simulink model "Ph3_2Lvl_SVPWM_Comparison"  (R2022b)
settings: Solver=FixedStepDiscrete  StartTime=0.0  StopTime=1.2  FixedStep=1/(100*9600)  RelTol=1e-3
libraries: spsSeriesRLCBranchLib x15, spsRMSLib x10, spsMosfetLib x6, simulink x5, spsThreePhaseVIMeasurementLib x2, spsDCVoltageSourceLib x1, spsGroundLib x1, spsVoltageMeasurementLib x1, sps_lib x1
settings Model: Creator=XIAO  LastModifiedBy=XIAO
settings SolverCC: AutoInsertRateTranBlk=on
settings DataIOCC: ReturnWorkspaceOutputs=off  LoggingToFile=on

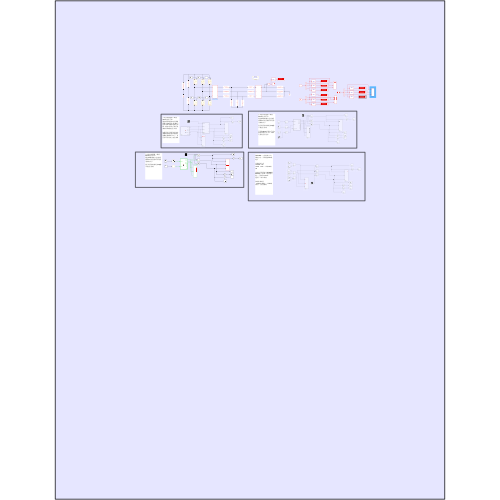
[thumbnail: Simulink's stored preview of the top-level diagram]
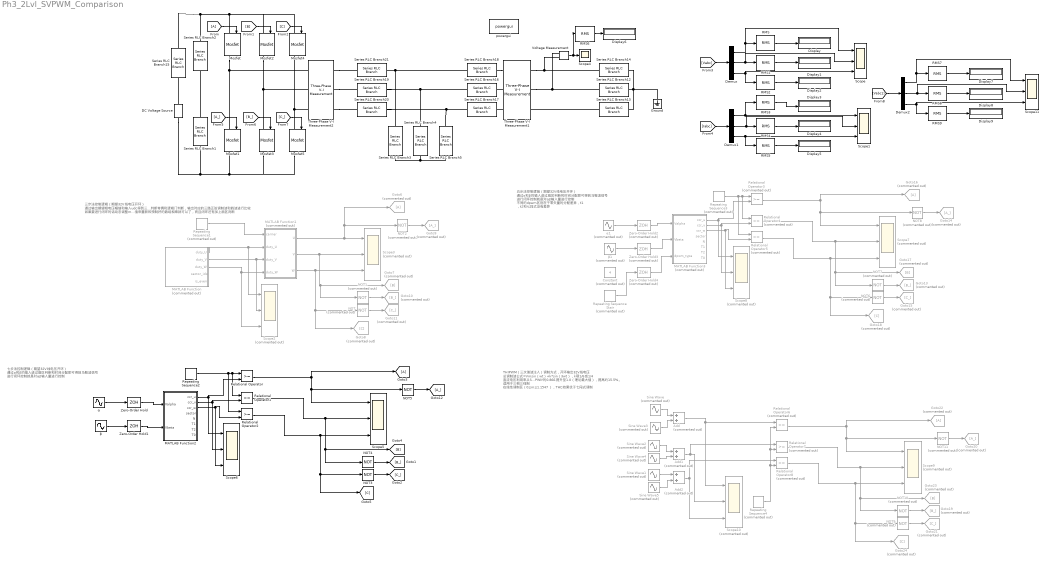
== system Ph3_2Lvl_SVPWM_Comparison ==
  note: 三步法控制逻辑（期望32V线电压开环）
      | 通过输出期望相电压幅值和输入udc得到三组数组，然后判断奇偶和逻辑门判断，输出对应的三路正弦调制波和载波进行比较
      |
      | 如果要进行闭环的话动态调整m值来重新和预制好的数组相乘就可以了，而且闭环还有加上扇区判断
  note: 七步法控制逻辑（期望32V线电压开环）
      | 通过α和β的输入进过扇区判断和时间分配即可得到马鞍波信号
      |
      | 进行闭环控制就是对αβ输入量进行控制
  note: 五步法控制逻辑（期望32V线电压开环）
      | 通过α和β的输入进过扇区判断和时间分配即可得到马鞍波信号
      |
      | 进行闭环控制就是对αβ输入量进行控制
      |
      | 不同的dpwm区别在于零矢量的分配差异，t1 ，t2和七段式没有差异
  note: THIPWM（三次谐波注入）调制方式，开环输出32V线电压
      |
      | 总调制波公式=Vmsin（wt）+k*sin（3wt），k取1/6或1/4
      |
      | 直流电压利用率从SPWM的0.866提升至1.0（理论最大值），提高约15.5%。
      | 适用于三相三线制
      |
      | 在线性调制区（0≤m≤1.1547），THD效果优于七段式调制
  Add : Sum  Commented=on
  Add1 : Sum  Commented=on
  Add2 : Sum  Commented=on
  Constant : Constant  Commented=on  Value=4
  DC Voltage Source : spsDCVoltageSourceLib/DC Voltage Source  Amplitude=60  Measurements=None
  Demux : Demux  Outputs=3
  Demux1 : Demux  Outputs=3
  Demux2 : Demux  Outputs=3
  Display{,1..9} (10 alike) : Display
  From : From
  Goto10 : Goto  Commented=on  GotoTag=B_
  Goto11 : Goto  Commented=on  GotoTag=C_
  Goto13 : Goto  Commented=on  GotoTag=B_
  Goto14 : Goto  Commented=on  GotoTag=A_
  Goto15 : Goto  Commented=on  GotoTag=C_
  Goto16 : Goto  Commented=on
  Goto17 : Goto  Commented=on  GotoTag=B
  Goto18 : Goto  Commented=on  GotoTag=C
  Goto19 : Goto  Commented=on  GotoTag=B_
  Goto20 : Goto  Commented=on  GotoTag=A_
  Goto21 : Goto  Commented=on  GotoTag=C_
  Goto22 : Goto  Commented=on
  Goto23 : Goto  Commented=on  GotoTag=B
  Goto24 : Goto  Commented=on  GotoTag=C
  Goto3 : Goto
  Goto6 : Goto  Commented=on
  Goto7 : Goto  Commented=on  GotoTag=B
  Goto8 : Goto  Commented=on  GotoTag=C
  Goto9 : Goto  Commented=on  GotoTag=A_
  Ground : spsGroundLib/Ground  LConnTagsString=a
  MATLAB Function : MATLAB Function  Commented=on  TreatAsAtomicUnit=on  SystemSampleTime=1/9600
  MATLAB Function1 : MATLAB Function  Commented=on  TreatAsAtomicUnit=on  SystemSampleTime=1/(100*9600)
  MATLAB Function2 : MATLAB Function  TreatAsAtomicUnit=on
  MATLAB Function3 : MATLAB Function  Commented=on  TreatAsAtomicUnit=on
  Mosfet{,1..5} (6 alike) : spsMosfetLib/Mosfet  Ron=0.1  Lon=0  Rd=0.01  Vfd=0  IC=0  Rs=1e5  Cs=inf  Measurements=on
  NOT{,1..2,6..11} (9 alike) : Logic  Commented=on  Operator=NOT  IconShape=distinctive  AllPortsSameDT=off  OutDataTypeStr=boolean
  NOT3 : Logic  Operator=NOT  IconShape=distinctive  AllPortsSameDT=off  OutDataTypeStr=boolean
  NOT4 : Logic  Operator=NOT  IconShape=distinctive  AllPortsSameDT=off  OutDataTypeStr=boolean
  NOT5 : Logic  Operator=NOT  IconShape=distinctive  AllPortsSameDT=off  OutDataTypeStr=boolean
  RMS{,1..9} (10 alike) : spsRMSLib/RMS  TrueRMS=on  Freq=50  RMSInit=120  Ts=1/(100*9600)
  Relational Operator : RelationalOperator  OutDataTypeStr=boolean  RndMeth=Simplest  InputSameDT=off
  Relational Operator1 : RelationalOperator  OutDataTypeStr=boolean  RndMeth=Simplest  InputSameDT=off
  Relational Operator2 : RelationalOperator  OutDataTypeStr=boolean  RndMeth=Simplest  InputSameDT=off
  Relational Operator{3..8} (6 alike) : RelationalOperator  Commented=on  OutDataTypeStr=boolean  RndMeth=Simplest  InputSameDT=off
  Repeating Sequence Stair : simulink/Sources/Repeating Sequence Stair  Commented=on  OutValues=[1 2 3 4 5 6]  tsamp=0.2  OutMin=[]  OutMax=[]  OutDataTypeStr=double  OutputDataTypeScalingMode=double  OutDataType=fixdt(0,8)  ConRadixGroup=Best Precision: Vector-wise  OutScaling=2^-12
  Repeating Sequence1 : simulink/Sources/Repeating Sequence  Commented=on  rep_seq_t=[0, 1/9600]  rep_seq_y=[0,1]
  Repeating Sequence2 : simulink/Sources/Repeating Sequence  rep_seq_t=[0, 1/20000, 1/10000]  rep_seq_y=[0,8500,0]
  Repeating Sequence3 : simulink/Sources/Repeating Sequence  Commented=on  rep_seq_t=[0, 1/20000, 1/10000]  rep_seq_y=[0,8500,0]
  Repeating Sequence4 : simulink/Sources/Repeating Sequence  Commented=on  rep_seq_t=[0, 1/20000, 1/10000]  rep_seq_y=[-1,1,-1]
  Scope{,1,5..6,11} (5 alike) : Scope  NumInputPorts=3
  Scope{2..3,7..10} (6 alike) : Scope  Commented=on  NumInputPorts=3
  Scope4 : Scope
  Series RLC Branch1 : spsSeriesRLCBranchLib/Series RLC Branch  LConnTagsString=__new0  RConnTagsString=__new0  BranchType=C  Resistance=1  Inductance=1e-3  SetiL0=off  InitialCurrent=0  Capacitance=1000e-6  Setx0=off  InitialVoltage=0  Measurements=None
  Series RLC Branch12 : spsSeriesRLCBranchLib/Series RLC Branch  LConnTagsString=__new0  RConnTagsString=__new0  BranchType=R  Resistance=200  Inductance=1e-3  SetiL0=off  InitialCurrent=0  Capacitance=1000e-6  Setx0=off  InitialVoltage=0  Measurements=None
  Series RLC Branch13 : spsSeriesRLCBranchLib/Series RLC Branch  LConnTagsString=__new0  RConnTagsString=__new0  BranchType=R  Resistance=200  Inductance=1e-3  SetiL0=off  InitialCurrent=0  Capacitance=1000e-6  Setx0=off  InitialVoltage=0  Measurements=None
  Series RLC Branch14 : spsSeriesRLCBranchLib/Series RLC Branch  LConnTagsString=__new0  RConnTagsString=__new0  BranchType=R  Resistance=200  Inductance=1e-3  SetiL0=off  InitialCurrent=0  Capacitance=1000e-6  Setx0=off  InitialVoltage=0  Measurements=None
  Series RLC Branch15 : spsSeriesRLCBranchLib/Series RLC Branch  LConnTagsString=__new0  RConnTagsString=__new0  BranchType=R  Resistance=0.1  Inductance=1e-3  SetiL0=off  InitialCurrent=0  Capacitance=1000e-6  Setx0=off  InitialVoltage=0  Measurements=None
  Series RLC Branch16 : spsSeriesRLCBranchLib/Series RLC Branch  LConnTagsString=__new0  RConnTagsString=__new0  BranchType=L  Resistance=1  Inductance=120.e-6  SetiL0=off  InitialCurrent=0  Capacitance=1000e-6  Setx0=off  InitialVoltage=0  Measurements=None
  Series RLC Branch17 : spsSeriesRLCBranchLib/Series RLC Branch  LConnTagsString=__new0  RConnTagsString=__new0  BranchType=L  Resistance=1  Inductance=120e-6  SetiL0=off  InitialCurrent=0  Capacitance=1000e-6  Setx0=off  InitialVoltage=0  Measurements=None
  Series RLC Branch18 : spsSeriesRLCBranchLib/Series RLC Branch  LConnTagsString=__new0  RConnTagsString=__new0  BranchType=L  Resistance=1  Inductance=120e-6  SetiL0=off  InitialCurrent=0  Capacitance=1000e-6  Setx0=off  InitialVoltage=0  Measurements=None
  Series RLC Branch19 : spsSeriesRLCBranchLib/Series RLC Branch  LConnTagsString=__new0  RConnTagsString=__new0  BranchType=L  Resistance=1  Inductance=1.5e-3  SetiL0=off  InitialCurrent=0  Capacitance=1000e-6  Setx0=off  InitialVoltage=0  Measurements=None
  Series RLC Branch2 : spsSeriesRLCBranchLib/Series RLC Branch  LConnTagsString=__new0  RConnTagsString=__new0  BranchType=C  Resistance=1  Inductance=1e-3  SetiL0=off  InitialCurrent=0  Capacitance=1000e-6  Setx0=off  InitialVoltage=0  Measurements=None
  Series RLC Branch20 : spsSeriesRLCBranchLib/Series RLC Branch  LConnTagsString=__new0  RConnTagsString=__new0  BranchType=L  Resistance=1  Inductance=1.5e-3  SetiL0=off  InitialCurrent=0  Capacitance=1000e-6  Setx0=off  InitialVoltage=0  Measurements=None
  Series RLC Branch21 : spsSeriesRLCBranchLib/Series RLC Branch  LConnTagsString=__new0  RConnTagsString=__new0  BranchType=L  Resistance=1  Inductance=1.5e-3  SetiL0=off  InitialCurrent=0  Capacitance=1000e-6  Setx0=off  InitialVoltage=0  Measurements=None
  Series RLC Branch3 : spsSeriesRLCBranchLib/Series RLC Branch  LConnTagsString=__new0  RConnTagsString=__new0  BranchType=C  Resistance=1  Inductance=1e-3  SetiL0=off  InitialCurrent=0  Capacitance=10e-6  Setx0=off  InitialVoltage=0  Measurements=None
  Series RLC Branch4 : spsSeriesRLCBranchLib/Series RLC Branch  LConnTagsString=__new0  RConnTagsString=__new0  BranchType=C  Resistance=1  Inductance=1e-3  SetiL0=off  InitialCurrent=0  Capacitance=10e-6  Setx0=off  InitialVoltage=0  Measurements=None
  Series RLC Branch5 : spsSeriesRLCBranchLib/Series RLC Branch  LConnTagsString=__new0  RConnTagsString=__new0  BranchType=C  Resistance=1  Inductance=1e-3  SetiL0=off  InitialCurrent=0  Capacitance=10e-6  Setx0=off  InitialVoltage=0  Measurements=None
  Sine Wave : Sin  Commented=on  Amplitude=0.871  Frequency=100*pi  SampleTime=0
  Sine Wave1 : Sin  Commented=on  Amplitude=0.871  Frequency=100*pi  Phase=-4*pi/3  SampleTime=0
  Sine Wave2 : Sin  Commented=on  Amplitude=0.871  Frequency=100*pi  Phase=-2*pi/3  SampleTime=0
  Sine Wave3 : Sin  Commented=on  Amplitude=0.145  Frequency=300*pi  SampleTime=0
  Sine Wave4 : Sin  Commented=on  Amplitude=0.145  Frequency=300*pi  SampleTime=0
  Sine Wave5 : Sin  Commented=on  Amplitude=0.145  Frequency=300*pi  SampleTime=0
  Three-Phase V-I Measurement1 : spsThreePhaseVIMeasurementLib/Three-Phase V-I Measurement  VoltageMeasurement=phase-to-ground  SetLabelV=on  LabelV=Vabc  Vpu=off  VpuLL=off  CurrentMeasurement=yes  SetLabelI=on  LabelI=Iabc  Ipu=off  Pbase=100e6  Vbase=500e3  OutputType=Complex  PhasorSimulation=off  PSBequivalent=0
  Three-Phase V-I Measurement2 : spsThreePhaseVIMeasurementLib/Three-Phase V-I Measurement  VoltageMeasurement=phase-to-phase  SetLabelV=on  LabelV=Vabc1  Vpu=off  VpuLL=off  CurrentMeasurement=yes  SetLabelI=on  LabelI=Iabc1  Ipu=off  Pbase=100e6  Vbase=500e3  OutputType=Complex  PhasorSimulation=off  PSBequivalent=0
  Voltage Measurement : spsVoltageMeasurementLib/Voltage Measurement  PhasorSimulation=off  OutputType=Complex  PSBequivalent=0
  Zero-Order Hold : ZeroOrderHold  SampleTime=5e-5
  Zero-Order Hold1 : ZeroOrderHold  SampleTime=5e-5
  Zero-Order Hold2 : ZeroOrderHold  Commented=on  SampleTime=5e-5
  Zero-Order Hold3 : ZeroOrderHold  Commented=on  SampleTime=5e-5
  Zero-Order Hold4 : ZeroOrderHold  Commented=on  SampleTime=5e-5
  powergui : sps_lib/powergui  Priority=1  SimulationMode=Discrete  SampleTime=1/(100*9600)  frequency=60  Iterations=50  frequencyindice=0  Pbase=100e6  ErrMax=1e-4  UnitsV=kV  UnitsW=MW  buscounter=0  FunctionMessages=off  echomessages=off  EnableUseOfTLC=off  CurrentSourceSwitches=off  DisableSnubberDevices=off  DisableRonSwitches=off  DisableVfSwitches=off  DisplayEquations=off  AutomaticDiscreteSolvers=off  SolverType=Tustin/Backward Euler (TBE)  Interpol=off  ExternalGateDelay=off  methode=off  Ts=100  x0status=blocks  SPID=on  SwTol=0  HookPort=off  NonlinearTolerance=1e-4  nMaxIteration=100  ContinueOnMaxIteration=off  RestoreLinks=warning  ResistiveCurrentMeasurement=off  Frange=[0:2:500]  Ylog=off  Xlog=on  ShowGrid=off  save=off  variable=ZData  structure=0  ZoomFFT=off  StartTime=0.0  cycles=1  DisplayStyle=1  fundamental=60  FreqAxis=off  MaxFrequency=1000  frequencyindicesteady=1  RmsSteady=1  display=off
  α : Sin  Amplitude=26.13  Frequency=100*pi  SampleTime=0
  α1 : Sin  Commented=on  Amplitude=26.13  Frequency=100*pi  SampleTime=0
  β : Sin  Amplitude=26.13  Frequency=100*pi  Phase=pi/2  SampleTime=0
  β1 : Sin  Commented=on  Amplitude=26.13  Frequency=100*pi  Phase=pi/2  SampleTime=0
  wires:
  [Vabc] -> Demux/1
  Demux/3 -> Scope/3, RMS2/1
  Demux/2 -> Scope/2, RMS1/1
  Demux/1 -> RMS/1, Scope/1
  RMS/1 -> Display/1
  RMS1/1 -> Display1/1
  RMS2/1 -> Display2/1
  RMS4/1 -> Display4/1
  [Iabc] -> Demux1/1
  Demux1/1 -> RMS3/1, Scope1/1
  Demux1/2 -> Scope1/2, RMS4/1
  RMS5/1 -> Display5/1
  RMS3/1 -> Display3/1
  Demux1/3 -> Scope1/3, RMS5/1
  Voltage Measurement/1 -> RMS6/1, Scope4/1
  From/1 -> Mosfet/1
  [B] -> Mosfet2/1
  [C] -> Mosfet4/1
  [C_] -> Mosfet5/1
  [B_] -> Mosfet3/1
  [A_] -> Mosfet1/1
  NOT/1 -> Goto11/1
  NOT1/1 -> Goto10/1
  NOT2/1 -> Goto9/1
  RMS6/1 -> Display6/1
  Repeating Sequence1/1 -> MATLAB Function1/1(carrier)
  MATLAB Function/1(duty_U) -> MATLAB Function1/2(duty_U), Scope2/1
  MATLAB Function/2(duty_V) -> Scope2/2, MATLAB Function1/3(duty_V)
  MATLAB Function/3(duty_W) -> Scope2/3, MATLAB Function1/4(duty_W)
  MATLAB Function1/1(U) -> Goto6/1, NOT2/1, Scope3/1
  MATLAB Function1/2(V) -> Scope3/2, NOT1/1, Goto7/1
  MATLAB Function1/3(W) -> Goto8/1, NOT/1, Scope3/3
  Relational Operator2/1 -> [C], NOT3/1, Scope5/3
  Relational Operator1/1 -> Scope5/2, NOT4/1, [B]
  NOT3/1 -> [C_]
  NOT5/1 -> [A_]
  NOT4/1 -> [B_]
  Zero-Order Hold/1 -> MATLAB Function2/1(Valpha)
  Zero-Order Hold1/1 -> MATLAB Function2/2(Vbeta)
  β/1 -> Zero-Order Hold1/1
  α/1 -> Zero-Order Hold/1
  Repeating Sequence2/1 -> Relational Operator2/1, Relational Operator1/1, Relational Operator/1
  MATLAB Function2/1(ccr_u) -> Relational Operator/2, Scope6/1
  MATLAB Function2/3(ccr_w) -> Scope6/3, Relational Operator2/2
  MATLAB Function2/2(ccr_v) -> Scope6/2, Relational Operator1/2
  Relational Operator/1 -> Goto3/1, Scope5/1, NOT5/1
  Relational Operator3/1 -> Goto16/1, Scope7/1, NOT8/1
  MATLAB Function3/3(ccr_w) -> Scope8/3, Relational Operator5/2
  Zero-Order Hold3/1 -> MATLAB Function3/2(Vbeta)
  Relational Operator5/1 -> Goto18/1, NOT6/1, Scope7/3
  β1/1 -> Zero-Order Hold3/1
  Relational Operator4/1 -> Scope7/2, NOT7/1, Goto17/1
  MATLAB Function3/1(ccr_u) -> Relational Operator3/2, Scope8/1
  α1/1 -> Zero-Order Hold2/1
  Repeating Sequence3/1 -> Relational Operator5/1, Relational Operator4/1, Relational Operator3/1
  Zero-Order Hold2/1 -> MATLAB Function3/1(Valpha)
  MATLAB Function3/2(ccr_v) -> Scope8/2, Relational Operator4/2
  NOT8/1 -> Goto14/1
  NOT6/1 -> Goto15/1
  NOT7/1 -> Goto13/1
  Zero-Order Hold4/1 -> MATLAB Function3/3(dpwm_type)
  Repeating Sequence Stair/1 -> Zero-Order Hold4/1
  NOT10/1 -> Goto19/1
  NOT9/1 -> Goto21/1
  Relational Operator6/1 -> Goto22/1, Scope9/1, NOT11/1
  Relational Operator7/1 -> Scope9/2, NOT10/1, Goto23/1
  NOT11/1 -> Goto20/1
  Relational Operator8/1 -> Goto24/1, NOT9/1, Scope9/3
  Sine Wave/1 -> Add/1
  Sine Wave3/1 -> Add/2
  Sine Wave2/1 -> Add1/1
  Sine Wave4/1 -> Add1/2
  Sine Wave1/1 -> Add2/1
  Sine Wave5/1 -> Add2/2
  Add/1 -> Relational Operator6/1, Scope10/1
  Add1/1 -> Relational Operator7/1, Scope10/2
  Add2/1 -> Relational Operator8/1, Scope10/3
  Repeating Sequence4/1 -> Relational Operator6/2, Relational Operator7/2, Relational Operator8/2
  RMS8/1 -> Display8/1
  RMS9/1 -> Display9/1
  [Vabc1] -> Demux2/1
  Demux2/2 -> Scope11/2, RMS8/1
  RMS7/1 -> Display7/1
  Demux2/1 -> RMS7/1, Scope11/1
  Demux2/3 -> Scope11/3, RMS9/1
  connections:
  Mosfet4/LConn1 -- Mosfet2/LConn1 -- Mosfet/LConn1 -- Series RLC Branch15/RConn1 -- Series RLC Branch2/LConn1
  Series RLC Branch3/RConn1 -- Series RLC Branch5/RConn1 -- Series RLC Branch4/RConn1
  DC Voltage Source/LConn1 -- Mosfet5/RConn1 -- Mosfet3/RConn1 -- Mosfet1/RConn1 -- Series RLC Branch1/RConn1
  Mosfet/RConn1 -- Mosfet1/LConn1 -- Three-Phase V-I Measurement2/LConn1
  Series RLC Branch1/LConn1 -- Series RLC Branch2/RConn1
  DC Voltage Source/RConn1 -- Series RLC Branch15/LConn1
  Three-Phase V-I Measurement1/RConn1 -- Series RLC Branch14/RConn1 -- Voltage Measurement/LConn2
  Three-Phase V-I Measurement1/RConn2 -- Series RLC Branch12/RConn1 -- Voltage Measurement/LConn1
  Series RLC Branch13/RConn1 -- Three-Phase V-I Measurement1/RConn3
  Series RLC Branch14/LConn1 -- Series RLC Branch12/LConn1 -- Ground/LConn1 -- Series RLC Branch13/LConn1
  Three-Phase V-I Measurement1/LConn2 -- Series RLC Branch16/LConn1
  Mosfet5/LConn1 -- Mosfet4/RConn1 -- Three-Phase V-I Measurement2/LConn3
  Mosfet2/RConn1 -- Three-Phase V-I Measurement2/LConn2 -- Mosfet3/LConn1
  Series RLC Branch18/LConn1 -- Three-Phase V-I Measurement1/LConn1
  Series RLC Branch20/LConn1 -- Series RLC Branch17/RConn1 -- Series RLC Branch5/LConn1
  Series RLC Branch19/LConn1 -- Series RLC Branch16/RConn1 -- Series RLC Branch4/LConn1
  Three-Phase V-I Measurement1/LConn3 -- Series RLC Branch17/LConn1
  Series RLC Branch3/LConn1 -- Series RLC Branch21/LConn1 -- Series RLC Branch18/RConn1
  Three-Phase V-I Measurement2/RConn1 -- Series RLC Branch21/RConn1
  Three-Phase V-I Measurement2/RConn2 -- Series RLC Branch19/RConn1
  Three-Phase V-I Measurement2/RConn3 -- Series RLC Branch20/RConn1

== matlab function Ph3_2Lvl_SVPWM_Comparison/MATLAB Function2 ==
  data: Valpha input; ccr_u output; Vbeta input; ccr_v output; ccr_w output; sector output; N output; T1 output; T2 output; T0 output
function [ccr_u,  ccr_v, ccr_w, sector, N, T1, T2, T0] = fcn( Valpha, Vbeta)
% #########################################################################
% 功能: 优化版两电平七段式SVPWM算法（采用XYZ法）
% 修正: 修复了增益系数缺失 sqrt3 以及扇区切换不连续导致的波形畸变
% 硬件对应: STM32G474 TIM1 中央对齐模式 (ARR=8500, 计数周期=2*ARR)
% #########################################################################

%% ===================== 1. 硬件及物理常量 =====================
persistent sqrt3 Udc ARR EPS
if isempty(sqrt3)
    sqrt3 = 1.732050807568877;
    Udc = 60.0;          % 母线电压
    ARR = 8500;          % 定时器自动重装载值
    EPS = 1e-6;          
end

%% ===================== 2. 零矢量提前判断 =====================
if abs(Valpha) + abs(Vbeta) < EPS
    sector = 0; N = 0; T1 = 0; T2 = 0; T0 = 2 * ARR;
    ccr_u = 4250; ccr_v = 4250; ccr_w = 4250;
    return;
end

%% ===================== 3. N因子法扇区判断 =====================
% 保持你的N因子逻辑，这是正确的
A = Vbeta;
B = (sqrt3/2) * Valpha - 0.5 * Vbeta;
C = -(sqrt3/2) * Valpha - 0.5 * Vbeta;

a = (A > 0);
b = (B > 0);
c = (C > 0);
N = a + 2*b + 4*c;

switch N
    case 3,  sector = 1;
    case 1,  sector = 2;
    case 5,  sector = 3;
    case 4,  sector = 4;
    case 6,  sector = 5;
    case 2,  sector = 6;
    otherwise, sector = 0;
end

%% ===================== 4. XYZ中间变量计算 =====================
% 核心修正：引入 sqrt3 增益补偿，提高电压利用率并修正波形比例
% K 因子包含了标准 SVPWM 推导中的 sqrt3 * Ts / Udc
K = sqrt3 * (ARR * 2.0) / Udc;

X = K * Vbeta;
Y = K * ( (sqrt3/2.0) * Valpha + 0.5 * Vbeta );
Z = K * ( -(sqrt3/2.0) * Valpha + 0.5 * Vbeta );

%% ===================== 5. 扇区矢量时间分配 =====================
T1 = 0.0; T2 = 0.0;
switch sector
    case 1, T1 = -Z; T2 = X;
    case 2, T1 = Z;  T2 = Y;
    case 3, T1 = X;  T2 = -Y;
    case 4, T1 = -X; T2 = Z;
    case 5, T1 = -Y; T2 = -Z;
    case 6, T1 = Y;  T2 = -X;
end

%% ===================== 6. 过调制处理 =====================
Tsum = T1 + T2;
if Tsum > 2.0 * ARR
    scale = (2.0 * ARR) / Tsum;
    T1 = T1 * scale;
    T2 = T2 * scale;
end
T0 = 2.0 * ARR - T1 - T2;

%% ===================== 7. 七段式切换点映射 =====================
% 定义三个基本切换时间点（半个PWM周期对称分配）
% Ta: 只有第一矢量和零矢量导通时的切换点
% Tb: 第二矢量加入后的切换点
% Tc: 进入全导通(V7)之前的切换点
t_p1 = T0 / 4.0;
t_p2 = t_p1 + T1 / 2.0;
t_p3 = t_p2 + T2 / 2.0;

% 根据扇区将这三个时间点分配给 U, V, W 相的 CCR 寄存器
% 注意：此处分配决定了波形的相位连续性，是解决“丑波形”的关键
switch sector
    case 1, ccr_u = t_p1; ccr_v = t_p2; ccr_w = t_p3; % V1, V2
    case 2, ccr_u = t_p2; ccr_v = t_p1; ccr_w = t_p3; % V3, V2
    case 3, ccr_u = t_p3; ccr_v = t_p1; ccr_w = t_p2; % V3, V4
    case 4, ccr_u = t_p3; ccr_v = t_p2; ccr_w = t_p1; % V5, V4
    case 5, ccr_u = t_p2; ccr_v = t_p3; ccr_w = t_p1; % V5, V6
    case 6, ccr_u = t_p1; ccr_v = t_p3; ccr_w = t_p2; % V1, V6
    otherwise
        ccr_u = 4250; ccr_v = 4250; ccr_w = 4250;
end

% 硬件数值处理：取整
ccr_u = round(ccr_u);
ccr_v = round(ccr_v);
ccr_w = round(ccr_w);

end

== matlab function Ph3_2Lvl_SVPWM_Comparison/MATLAB Function ==
  data: duty_U output; duty_V output; duty_W output; sector_idx output; is_even output
function [duty_U, duty_V, duty_W, sector_idx, is_even] = fcn()
% #########################################################################
% 功能: 模拟单片机 9.6kHz 定时器中断服务程序 (ISR)
% 任务: 
%   1. 维护奇偶调制周期与扇区状态机 [cite: 334]
%   2. 查表获取预先计算好的单位作用时间 (Pk, Pk+1, P0) [cite: 527]
%   3. 将论文中的组合逻辑方程 (表3-5) 映射为最终的占空比数值 [cite: 586]
% #########################################################################

% --- 静态内存变量 (模拟单片机全局变量) ---
persistent Qk Qk1 Q sample_cnt s_idx even_flag

if isempty(sample_cnt)
    % 预置内存数组 (n=32): 存储单位幅值直角锯齿波对调制波规则采样得到的值 [cite: 504, 526]
    % 这些数组对应论文中的 Pk, Pk+1, P0 (假设幅度系数 a=1) [cite: 497, 593]
    Qk  = [0.6469 0.6339 0.6202 0.6058 0.5908 0.5751 0.5589 0.5420 0.5245 0.5065 0.4880 0.4689 0.4493 0.4292 0.4087 0.3878 0.3664 0.3446 0.3225 0.3000 0.2772 0.2541 0.2307 0.2071 0.1833 0.1592 0.1350 0.1107 0.0862 0.0616 0.0370 0.0123];
    Qk1 = [0.0123 0.0370 0.0616 0.0862 0.1107 0.1350 0.1592 0.1833 0.2071 0.2307 0.2541 0.2772 0.3000 0.3225 0.3446 0.3664 0.3878 0.4087 0.4292 0.4493 0.4689 0.4880 0.5065 0.5245 0.5420 0.5589 0.5751 0.5908 0.6058 0.6202 0.6339 0.6469];
    Q   = [0.6593 0.6709 0.6818 0.6920 0.7015 0.7102 0.7181 0.7253 0.7316 0.7372 0.7421 0.7461 0.7493 0.7517 0.7533 0.7541 0.7541 0.7533 0.7517 0.7493 0.7461 0.7421 0.7372 0.7316 0.7253 0.7181 0.7102 0.7015 0.6920 0.6818 0.6709 0.6593];
    
    sample_cnt = 1.0; % 采样点计数器 (1~32)
    s_idx = 1.0;      % 扇区索引 (1~6) [cite: 541]
    even_flag = 0.0;  % 奇偶标志: 0代表奇调制周期，1代表偶调制周期 [cite: 559]
end

% --- 1. 状态更新 (时序控制) ---
% 翻转奇偶标志，实现 2Ts 长度的完整周期 [cite: 560]
even_flag = 1.0 - even_flag;

% 每完成一个奇偶循环 (即 even_flag 回到 0) 时，步进采样角度
if even_flag == 0.0
    sample_cnt = sample_cnt + 1.0;
    
    % 完成一个扇区的采样后，切换到下一扇区 [cite: 541]
    if sample_cnt > 32.0
        sample_cnt = 1.0;
        s_idx = s_idx + 1.0;
        % 六个扇区循环往复 [cite: 206, 555]
        if s_idx > 6.0, s_idx = 1.0; end
    end
end

% --- 2. 查表获取当前时刻的作用时间 ---
idx = int32(sample_cnt);
rQ   = Q(idx);   % P0 (零矢量与基本矢量总占比)
rQk  = Qk(idx);  % Pk (基本矢量k占比)
rQk1 = Qk1(idx); % Pk+1 (基本矢量k+1占比)

% --- 3. 逻辑预处理 -> 映射为占空比数值 ---
% 本段将论文表 3-5 中的布尔方程转化为数值运算 [cite: 585, 586]
% 映射原理：
%   逻辑 1 (恒高) -> 占空比数值 0.0 (CCR=0 对应全周期 Carrier > CCR)
%   逻辑 T0_L (Carrier > rQ) -> 占空比数值 rQ
%   或门 (|) -> 取最小值 min()。因为阈值越小，Carrier > CCR 的覆盖范围越大
%   非门 (~) -> 1.0 减去原值 [cite: 586]

d_u = 0.0; d_v = 0.0; d_w = 0.0;
cur_s = int32(s_idx);

if even_flag == 0.0
    % --- 奇数状态逻辑 (奇调制波, 最后一个矢量为 U7(111)) [cite: 472, 478] ---
    switch cur_s
        case 1, d_u=0.0;           d_v=min(rQ, rQk);  d_w=rQ;             % U=1, V=T0|~Tk, W=T0
        case 2, d_u=min(rQ, rQk1); d_v=0.0;           d_w=rQ;             % U=T0|~Tk1, V=1, W=T0
        case 3, d_u=rQ;            d_v=0.0;           d_w=min(rQ, rQk);   % U=T0, V=1, W=T0|~Tk
        case 4, d_u=rQ;            d_v=min(rQ, rQk1); d_w=0.0;            % U=T0, V=T0|~Tk1, W=1
        case 5, d_u=min(rQ, rQk);  d_v=rQ;            d_w=0.0;            % U=T0|~Tk, V=T0, W=1
        case 6, d_u=0.0;           d_v=rQ;            d_w=min(rQ, rQk1);  % U=1, V=T0, W=T0|~Tk1
    end
else
    % --- 偶数状态逻辑 (偶调制波, 最后一个矢量为 U0(000)) [cite: 472, 478] ---
    % 偶周期逻辑多为 ~T0&Tk 形式，映射为 1-X 结构
    switch cur_s
        case 1, d_u=1.0-rQ;        d_v=1.0-min(rQ, rQk1); d_w=1.0;        % U=~T0, V=~T0&Tk1, W=0
        case 2, d_u=1.0-min(rQ, rQk); d_v=1.0-rQ;         d_w=1.0;        % U=~T0&Tk, V=~T0, W=0
        case 3, d_u=1.0;           d_v=1.0-rQ;            d_w=1.0-min(rQ, rQk1); % U=0, V=~T0, W=~T0&Tk1
        case 4, d_u=1.0;           d_v=1.0-min(rQ, rQk);  d_w=1.0-rQ;     % U=0, V=~T0&Tk, W=~T0
        case 5, d_u=1.0-min(rQ, rQk1); d_v=1.0;           d_w=1.0-rQ;     % U=~T0&Tk1, V=0, W=~T0
        case 6, d_u=1.0-rQ;        d_v=1.0;               d_w=1.0-min(rQ, rQk);  % U=~T0, V=0, W=~T0&Tk
    end
end

% --- 4. 赋值输出 ---
% duty_X 范围 0.0~1.0，直接作为硬件 PWM 的比较阈值
duty_U = d_u; 
duty_V = d_v; 
duty_W = d_w;
sector_idx = s_idx;
is_even = even_flag;

end

== matlab function Ph3_2Lvl_SVPWM_Comparison/MATLAB Function3 ==
  data: Valpha input; ccr_u output; Vbeta input; ccr_v output; ccr_w output; sector output; N output; T1 output; T2 output; T0 output; dpwm_type input
function [ccr_u,  ccr_v, ccr_w, sector, N, T1, T2, T0] = fcn( Valpha, Vbeta, dpwm_type)
% #########################################################################
% 功能: 兼容 6 种全系列 DPWM 调制算法的统一硬件映射函数
% 输入: Valpha, Vbeta - 控制电压; dpwm_type - 模式选择 (1~6)
% 硬件对应: STM32G474 TIM1 中央对齐模式 (ARR=8500, 计数周期=2*ARR)
% #########################################################################
%% ===================== 1. 硬件及物理常量 =====================
persistent sqrt3 Udc ARR EPS
if isempty(sqrt3)
    sqrt3 = 1.732050807568877;
    Udc = 60.0;          % 母线电压
    ARR = 8500;          % 定时器自动重装载值
    EPS = 1e-6;          
end

%% ===================== 2. 零矢量提前判断 =====================
if abs(Valpha) + abs(Vbeta) < EPS
    sector = 0; N = 0; T1 = 0; T2 = 0; T0 = 2 * ARR;
    ccr_u = 4250; ccr_v = 4250; ccr_w = 4250;
    return;
end

%% ===================== 3. N因子法标准大扇区判断 (1~6) =====================
A = Vbeta;
B = (sqrt3/2) * Valpha - 0.5 * Vbeta;
C = -(sqrt3/2) * Valpha - 0.5 * Vbeta;
a = (A > 0);
b = (B > 0);
c = (C > 0);
N = a + 2*b + 4*c;
switch N
    case 3,  sector = 1;
    case 1,  sector = 2;
    case 5,  sector = 3;
    case 4,  sector = 4;
    case 6,  sector = 5;
    case 2,  sector = 6;
    otherwise, sector = 0;
end

%% ===================== 4. 12个细分小扇区判断 (用于 DPWM1 和 DPWM3) =====================
% 计算电压矢量的绝对角度 theta，范围 [0, 2*pi)
theta = atan2(Vbeta, Valpha);
if theta < 0
    theta = theta + 2.0 * 3.141592653589793;
end
theta_deg = theta * 180.0 / 3.141592653589793;

% 每 30° 为一个小扇区，共 1~12 个小扇区
% 注：大扇区 1 对应小扇区 1(0°-30°) 和 2(30°-60°)，以此类推
sub_sector = floor(theta_deg / 30.0) + 1;
if sub_sector > 12
    sub_sector = 12;
end

%% ===================== 5. XYZ中间变量及大扇区时间分配 =====================
K = sqrt3 * (ARR * 2.0) / Udc;
X = K * Vbeta;
Y = K * ( (sqrt3/2.0) * Valpha + 0.5 * Vbeta );
Z = K * ( -(sqrt3/2.0) * Valpha + 0.5 * Vbeta );

T1 = 0.0; T2 = 0.0;
switch sector
    case 1, T1 = -Z; T2 = X;
    case 2, T1 = Z;  T2 = Y;
    case 3, T1 = X;  T2 = -Y;
    case 4, T1 = -X; T2 = Z;
    case 5, T1 = -Y; T2 = -Z;
    case 6, T1 = Y;  T2 = -X;
end

%% ===================== 6. 过调制处理 =====================
Tsum = T1 + T2;
if Tsum > 2.0 * ARR
    scale = (2.0 * ARR) / Tsum;
    T1 = T1 * scale;
    T2 = T2 * scale;
end
T0 = 2.0 * ARR - T1 - T2;

%% ===================== 7. 6种 DPWM 核心零矢量选择逻辑 =====================
% 初始化选择：false -> 选用 V0 (籍位到负母线); true -> 选用 V7 (籍位到正母线)
use_v7 = false; 

switch dpwm_type
    case 1  % 【DPWMMIN】 固定选用零矢量 v0
        use_v7 = false;
        
    case 2  % 【DPWMMAX】 固定选用零矢量 v7
        use_v7 = true;
        
    case 3  % 【DPWM0】 1,2,4 扇区选 v7；3,5,6 扇区选 v0
        if (sector == 1 || sector == 2 || sector == 4)
            use_v7 = true;
        else
            use_v7 = false;
        end
        
    case 4  % 【DPWM1】 以基本矢量 u1(0°), u2(120°), u4(240°) 为中心的 60° 区域选 v7，其余选 v0
            % 对应小扇区：[330°~30°](12,1), [90°~150°](4,5), [210°~270°](8,9)
        if (sub_sector == 12 || sub_sector == 1 || sub_sector == 4 || ...
            sub_sector == 5  || sub_sector == 8 || sub_sector == 9)
            use_v7 = true;
        else
            use_v7 = false;
        end
        
    case 5  % 【DPWM2】 1,2,4 扇区选 v0；3,5,6 扇区选 v7 （与 DPWM0 互补）
        if (sector == 3 || sector == 5 || sector == 6)
            use_v7 = true;
        else
            use_v7 = false;
        end
        
    case 6  % 【DPWM3】 12小扇区交替。依据文献定义，刚好与 DPWM1 的零矢量选择相反
        if (sub_sector == 12 || sub_sector == 1 || sub_sector == 4 || ...
            sub_sector == 5  || sub_sector == 8 || sub_sector == 9)
            use_v7 = false;
        else
            use_v7 = true;
        end
end

%% ===================== 8. 计算五段式时间基准点 =====================
if use_v7
    % 籍位到 P 电平 (最高电压相全导通，CCR = 0)
    t_p1 = 0.0;
    t_p2 = T1 / 2.0;
    t_p3 = t_p2 + T2 / 2.0;
else
    % 籍位到 N 电平 (最低电压相全关闭，CCR = ARR)
    t_p1 = T0 / 2.0;
    t_p2 = t_p1 + T1 / 2.0;
    t_p3 = ARR; 
end

%% ===================== 9. 传统大扇区到硬件 CCR 的映射 =====================
switch sector
    case 1, ccr_u = t_p1; ccr_v = t_p2; ccr_w = t_p3; % V1, V2
    case 2, ccr_u = t_p2; ccr_v = t_p1; ccr_w = t_p3; % V3, V2
    case 3, ccr_u = t_p3; ccr_v = t_p1; ccr_w = t_p2; % V3, V4
    case 4, ccr_u = t_p3; ccr_v = t_p2; ccr_w = t_p1; % V5, V4
    case 5, ccr_u = t_p2; ccr_v = t_p3; ccr_w = t_p1; % V5, V6
    case 6, ccr_u = t_p1; ccr_v = t_p3; ccr_w = t_p2; % V1, V6
    otherwise
        ccr_u = 4250; ccr_v = 4250; ccr_w = 4250;
end

% 硬件数值取整
ccr_u = round(ccr_u);
ccr_v = round(ccr_v);
ccr_w = round(ccr_w);
end

== matlab function Ph3_2Lvl_SVPWM_Comparison/MATLAB Function1 ==
  data: carrier input; U output; duty_U input; duty_V input; duty_W input; V output; W output
function [U, V, W] = fcn(carrier, duty_U, duty_V, duty_W)
% #########################################################################
% 功能: 模拟硬件 PWM 比较器 (高频运行，如 1MHz 或更高)
% 输入: carrier (0~1 之间的锯齿波或三角波)
%      duty_U, duty_V, duty_W (来自 9.6kHz 中断计算出的比较阈值)
% #########################################################################

% 核心比较逻辑：
% 如果载波当前值大于阈值，输出高电平 (1)；否则输出低电平 (0)。
% 这是单片机硬件生成 PWM 波的最基本物理过程。

U = double(carrier > duty_U);
V = double(carrier > duty_V);
W = double(carrier > duty_W);

end
